simulink library "gm_ADC_Capture_4x4_IQ_DDR4_lib"  (R2019b)
settings: Solver=VariableStepAuto  StartTime=0.0  StopTime=10.0  RelTol=1e-3
undefined symbols (not defined in the file or in its folder): AXI4, Lite
libraries: axiinterfacelib x27
settings Model: Creator=larry  LastModifiedBy=larry

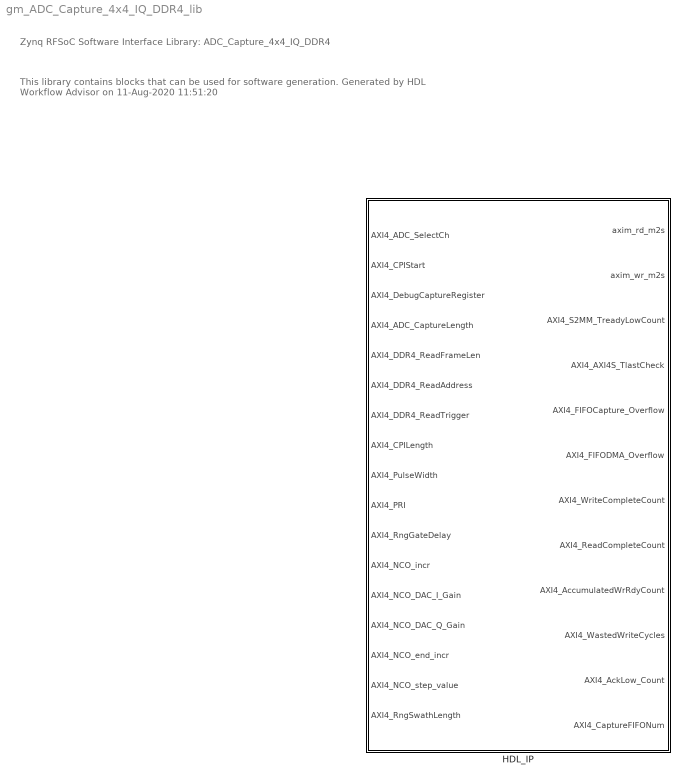
== system gm_ADC_Capture_4x4_IQ_DDR4_lib ==
  note: Zynq RFSoC Software Interface Library: ADC_Capture_4x4_IQ_DDR4
  note: This library contains blocks that can be used for software generation.
      |
      | Generated by HDL Workflow Advisor on 11-Aug-2020 11:51:20
  HDL_IP : Subsystem  TreatAsAtomicUnit=on  mask(AXI4-Lite/AXI4 Interface){}
      mask help:
      | This is an automatically generated subsystem block.
      | This contains the AXI interface blocks that communicate with the HDL_IP_ip IPCore generated from ADC_Capture_4x4_IQ_DDR4/HDL_IP subsystem.
      mask Display: disp(sprintf('Xilinx Zynq \nAXI Interface'));

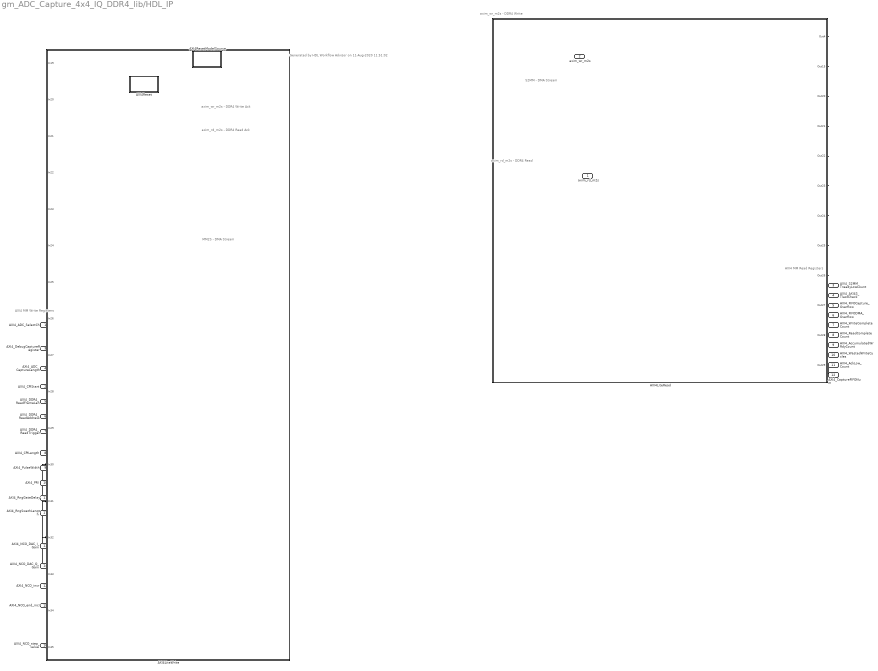
== system gm_ADC_Capture_4x4_IQ_DDR4_lib/HDL_IP ==
  note: Generated by HDL Workflow Advisor on 11-Aug-2020 11:51:02
  note: MM2S - DMA Stream
  note: axim_wr_m2s - DDR4 Write
  note: axim_rd_m2s - DDR4 Read Ack
  note: axim_rd_m2s - DDR4 Read
  note: axim_wr_m2s - DDR4 Write Ack
  note: S2MM - DMA Stream
  note: AXI4 MM Write Registers
  note: AXI4 MM Read Registers
  AXI4_ADC_SelectCh : Inport
  AXI4_CPIStart : Inport  Port=2
  AXI4_DebugCaptureRegister : Inport  Port=3
  AXI4_ADC_CaptureLength : Inport  Port=4
  AXI4_DDR4_ReadFrameLen : Inport  Port=5
  AXI4_DDR4_ReadAddress : Inport  Port=6
  AXI4_DDR4_ReadTrigger : Inport  Port=7
  AXI4_CPILength : Inport  Port=8
  AXI4_PulseWidth : Inport  Port=9
  AXI4_PRI : Inport  Port=10
  AXI4_RngGateDelay : Inport  Port=11
  AXI4_NCO_incr : Inport  Port=12
  AXI4_NCO_DAC_I_Gain : Inport  Port=13
  AXI4_NCO_DAC_Q_Gain : Inport  Port=14
  AXI4_NCO_end_incr : Inport  Port=15
  AXI4_NCO_step_value : Inport  Port=16
  AXI4_RngSwathLength : Inport  Port=17
  AXI4LiteRead : Subsystem  Priority=10
  AXI4LiteWrite : Subsystem  Priority=1
  AXI4Reset : Subsystem  mask(System Start){ShowInLibBrowser=0}
      mask prompts: ShowInLibBrowser "Simulink:masks:CustCodeMaskParam1_MP"
      settings: CopyFcn=cccopyfcn(gcb)  OpenFcn=ccopenfcn('System Start Function')
      mask Help: eval('feval(''rtwprivate'',''rtwhelpview'',''rtw_sys_start_block'')');
      mask Display: disp('System\nStart');
  AXI4ResetModelSource : Subsystem  mask(Model Source){ShowInLibBrowser=0}
      mask prompts: ShowInLibBrowser "Simulink:masks:CustCodeMaskParam1_MP"
      settings: CopyFcn=cccopyfcn(gcb)  OpenFcn=ccopenfcn('Model Source')
      mask Help: eval('feval(''rtwprivate'',''rtwhelpview'',''rtw_model_source_block'')');
      mask Display: disp('Model\nSource');
  axim_rd_m2s : Outport  VectorParamsAs1DForOutWhenUnconnected=off
  axim_wr_m2s : Outport  Port=2  VectorParamsAs1DForOutWhenUnconnected=off
  AXI4_S2MM_TreadyLowCount : Outport  Port=3  VectorParamsAs1DForOutWhenUnconnected=off
  AXI4_AXI4S_TlastCheck : Outport  Port=4  VectorParamsAs1DForOutWhenUnconnected=off
  AXI4_FIFOCapture_Overflow : Outport  Port=5  VectorParamsAs1DForOutWhenUnconnected=off
  AXI4_FIFODMA_Overflow : Outport  Port=6  VectorParamsAs1DForOutWhenUnconnected=off
  AXI4_WriteCompleteCount : Outport  Port=7  VectorParamsAs1DForOutWhenUnconnected=off
  AXI4_ReadCompleteCount : Outport  Port=8  VectorParamsAs1DForOutWhenUnconnected=off
  AXI4_AccumulatedWrRdyCount : Outport  Port=9  VectorParamsAs1DForOutWhenUnconnected=off
  AXI4_WastedWriteCycles : Outport  Port=10  VectorParamsAs1DForOutWhenUnconnected=off
  AXI4_AckLow_Count : Outport  Port=11  VectorParamsAs1DForOutWhenUnconnected=off
  AXI4_CaptureFIFONum : Outport  Port=12  VectorParamsAs1DForOutWhenUnconnected=off
  wires:
  AXI4LiteRead/12(Out29) -> AXI4_CaptureFIFONum/1
  AXI4LiteRead/11(Out28) -> AXI4_AckLow_Count/1
  AXI4LiteRead/10(Out27) -> AXI4_WastedWriteCycles/1
  AXI4LiteRead/9(Out26) -> AXI4_AccumulatedWrRdyCount/1
  AXI4LiteRead/8(Out25) -> AXI4_ReadCompleteCount/1
  AXI4LiteRead/7(Out24) -> AXI4_WriteCompleteCount/1
  AXI4LiteRead/6(Out23) -> AXI4_FIFODMA_Overflow/1
  AXI4LiteRead/5(Out22) -> AXI4_FIFOCapture_Overflow/1
  AXI4LiteRead/4(Out21) -> AXI4_AXI4S_TlastCheck/1
  AXI4LiteRead/3(Out20) -> AXI4_S2MM_TreadyLowCount/1
  AXI4LiteRead/2(Out15) -> axim_rd_m2s/1
  AXI4LiteRead/1(Out4) -> axim_wr_m2s/1
  AXI4_NCO_step_value/1 -> AXI4LiteWrite/17(In35)
  AXI4_NCO_end_incr/1 -> AXI4LiteWrite/16(In34)
  AXI4_NCO_incr/1 -> AXI4LiteWrite/15(In33)
  AXI4_NCO_DAC_Q_Gain/1 -> AXI4LiteWrite/14(In32)
  AXI4_NCO_DAC_I_Gain/1 -> AXI4LiteWrite/13(In31)
  AXI4_RngSwathLength/1 -> AXI4LiteWrite/12(In30)
  AXI4_RngGateDelay/1 -> AXI4LiteWrite/11(In29)
  AXI4_PRI/1 -> AXI4LiteWrite/10(In28)
  AXI4_PulseWidth/1 -> AXI4LiteWrite/9(In27)
  AXI4_CPILength/1 -> AXI4LiteWrite/8(In26)
  AXI4_DDR4_ReadTrigger/1 -> AXI4LiteWrite/7(In25)
  AXI4_DDR4_ReadAddress/1 -> AXI4LiteWrite/6(In24)
  AXI4_DDR4_ReadFrameLen/1 -> AXI4LiteWrite/5(In23)
  AXI4_CPIStart/1 -> AXI4LiteWrite/4(In22)
  AXI4_ADC_CaptureLength/1 -> AXI4LiteWrite/3(In21)
  AXI4_DebugCaptureRegister/1 -> AXI4LiteWrite/2(In20)
  AXI4_ADC_SelectCh/1 -> AXI4LiteWrite/1(In19)

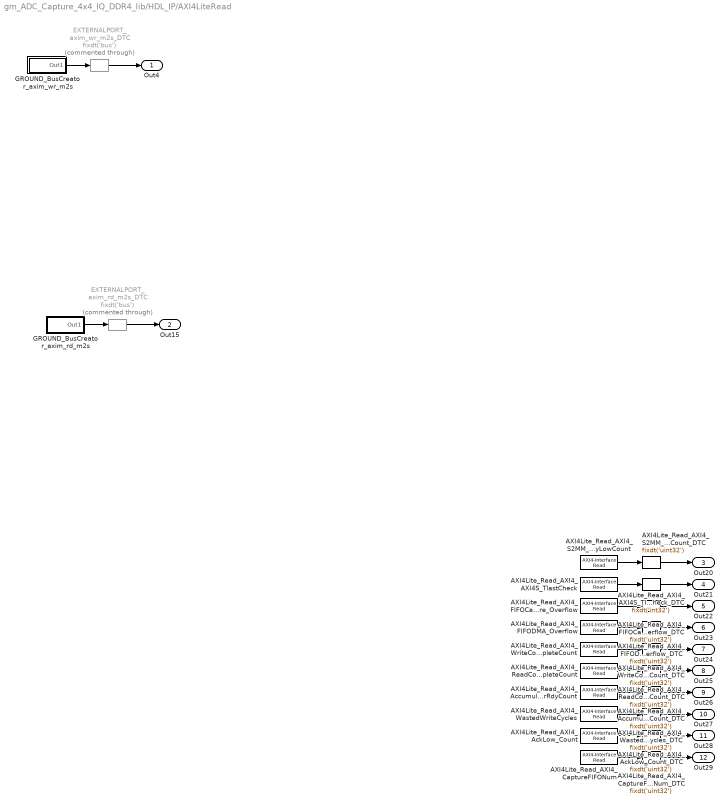
== system gm_ADC_Capture_4x4_IQ_DDR4_lib/HDL_IP/AXI4LiteRead ==
  AXI4Lite_Read_AXI4_AXI4S_TlastCheck : axiinterfacelib/AXI4-Interface Read  Priority=22  AXIInterfaceType=AXI4-Lite  DeviceName=/dev/mwipcore  RegisterOffset=hex2dec('148')  DataLength=1  DataType=uint32  SampleTime=-1  blockPlatform=ZYNQ  SimulateUsing=Interpreted Execution
      settings: SourceProductName=Embedded Coder Support Package for Xilinx Zynq Platform  SourceProductBaseCode=ECZYNQ7000
  AXI4Lite_Read_AXI4_AXI4S_TlastCheck_DTC : DataTypeConversion  OutDataTypeStr=fixdt('int32')  ConvertRealWorld=Stored Integer (SI)
  AXI4Lite_Read_AXI4_AccumulatedWrRdyCount : axiinterfacelib/AXI4-Interface Read  Priority=27  AXIInterfaceType=AXI4-Lite  DeviceName=/dev/mwipcore  RegisterOffset=hex2dec('15C')  DataLength=1  DataType=uint32  SampleTime=-1  blockPlatform=ZYNQ  SimulateUsing=Interpreted Execution
      settings: SourceProductName=Embedded Coder Support Package for Xilinx Zynq Platform  SourceProductBaseCode=ECZYNQ7000
  AXI4Lite_Read_AXI4_AccumulatedWrRdyCount_DTC : DataTypeConversion  OutDataTypeStr=fixdt('uint32')  ConvertRealWorld=Stored Integer (SI)
  AXI4Lite_Read_AXI4_AckLow_Count : axiinterfacelib/AXI4-Interface Read  Priority=29  AXIInterfaceType=AXI4-Lite  DeviceName=/dev/mwipcore  RegisterOffset=hex2dec('164')  DataLength=1  DataType=uint32  SampleTime=-1  blockPlatform=ZYNQ  SimulateUsing=Interpreted Execution
      settings: SourceProductName=Embedded Coder Support Package for Xilinx Zynq Platform  SourceProductBaseCode=ECZYNQ7000
  AXI4Lite_Read_AXI4_AckLow_Count_DTC : DataTypeConversion  OutDataTypeStr=fixdt('uint32')  ConvertRealWorld=Stored Integer (SI)
  AXI4Lite_Read_AXI4_CaptureFIFONum : axiinterfacelib/AXI4-Interface Read  Priority=30  AXIInterfaceType=AXI4-Lite  DeviceName=/dev/mwipcore  RegisterOffset=hex2dec('168')  DataLength=1  DataType=uint32  SampleTime=-1  blockPlatform=ZYNQ  SimulateUsing=Interpreted Execution
      settings: SourceProductName=Embedded Coder Support Package for Xilinx Zynq Platform  SourceProductBaseCode=ECZYNQ7000
  AXI4Lite_Read_AXI4_CaptureFIFONum_DTC : DataTypeConversion  OutDataTypeStr=fixdt('uint32')  ConvertRealWorld=Stored Integer (SI)
  AXI4Lite_Read_AXI4_FIFOCapture_Overflow : axiinterfacelib/AXI4-Interface Read  Priority=23  AXIInterfaceType=AXI4-Lite  DeviceName=/dev/mwipcore  RegisterOffset=hex2dec('14C')  DataLength=1  DataType=uint32  SampleTime=-1  blockPlatform=ZYNQ  SimulateUsing=Interpreted Execution
      settings: SourceProductName=Embedded Coder Support Package for Xilinx Zynq Platform  SourceProductBaseCode=ECZYNQ7000
  AXI4Lite_Read_AXI4_FIFOCapture_Overflow_DTC : DataTypeConversion  OutDataTypeStr=fixdt('uint32')  ConvertRealWorld=Stored Integer (SI)
  AXI4Lite_Read_AXI4_FIFODMA_Overflow : axiinterfacelib/AXI4-Interface Read  Priority=24  AXIInterfaceType=AXI4-Lite  DeviceName=/dev/mwipcore  RegisterOffset=hex2dec('150')  DataLength=1  DataType=uint32  SampleTime=-1  blockPlatform=ZYNQ  SimulateUsing=Interpreted Execution
      settings: SourceProductName=Embedded Coder Support Package for Xilinx Zynq Platform  SourceProductBaseCode=ECZYNQ7000
  AXI4Lite_Read_AXI4_FIFODMA_Overflow_DTC : DataTypeConversion  OutDataTypeStr=fixdt('uint32')  ConvertRealWorld=Stored Integer (SI)
  AXI4Lite_Read_AXI4_ReadCompleteCount : axiinterfacelib/AXI4-Interface Read  Priority=26  AXIInterfaceType=AXI4-Lite  DeviceName=/dev/mwipcore  RegisterOffset=hex2dec('158')  DataLength=1  DataType=uint32  SampleTime=-1  blockPlatform=ZYNQ  SimulateUsing=Interpreted Execution
      settings: SourceProductName=Embedded Coder Support Package for Xilinx Zynq Platform  SourceProductBaseCode=ECZYNQ7000
  AXI4Lite_Read_AXI4_ReadCompleteCount_DTC : DataTypeConversion  OutDataTypeStr=fixdt('uint32')  ConvertRealWorld=Stored Integer (SI)
  AXI4Lite_Read_AXI4_S2MM_TreadyLowCount : axiinterfacelib/AXI4-Interface Read  Priority=21  AXIInterfaceType=AXI4-Lite  DeviceName=/dev/mwipcore  RegisterOffset=hex2dec('144')  DataLength=1  DataType=uint32  SampleTime=-1  blockPlatform=ZYNQ  SimulateUsing=Interpreted Execution
      settings: SourceProductName=Embedded Coder Support Package for Xilinx Zynq Platform  SourceProductBaseCode=ECZYNQ7000
  AXI4Lite_Read_AXI4_S2MM_TreadyLowCount_DTC : DataTypeConversion  OutDataTypeStr=fixdt('uint32')  ConvertRealWorld=Stored Integer (SI)
  AXI4Lite_Read_AXI4_WastedWriteCycles : axiinterfacelib/AXI4-Interface Read  Priority=28  AXIInterfaceType=AXI4-Lite  DeviceName=/dev/mwipcore  RegisterOffset=hex2dec('160')  DataLength=1  DataType=uint32  SampleTime=-1  blockPlatform=ZYNQ  SimulateUsing=Interpreted Execution
      settings: SourceProductName=Embedded Coder Support Package for Xilinx Zynq Platform  SourceProductBaseCode=ECZYNQ7000
  AXI4Lite_Read_AXI4_WastedWriteCycles_DTC : DataTypeConversion  OutDataTypeStr=fixdt('uint32')  ConvertRealWorld=Stored Integer (SI)
  AXI4Lite_Read_AXI4_WriteCompleteCount : axiinterfacelib/AXI4-Interface Read  Priority=25  AXIInterfaceType=AXI4-Lite  DeviceName=/dev/mwipcore  RegisterOffset=hex2dec('154')  DataLength=1  DataType=uint32  SampleTime=-1  blockPlatform=ZYNQ  SimulateUsing=Interpreted Execution
      settings: SourceProductName=Embedded Coder Support Package for Xilinx Zynq Platform  SourceProductBaseCode=ECZYNQ7000
  AXI4Lite_Read_AXI4_WriteCompleteCount_DTC : DataTypeConversion  OutDataTypeStr=fixdt('uint32')  ConvertRealWorld=Stored Integer (SI)
  EXTERNALPORT_axim_rd_m2s_DTC : DataTypeConversion  Commented=through  OutDataTypeStr=fixdt('bus')
  EXTERNALPORT_axim_wr_m2s_DTC : DataTypeConversion  Commented=through  OutDataTypeStr=fixdt('bus')
  GROUND_BusCreator_axim_rd_m2s : Subsystem
  GROUND_BusCreator_axim_wr_m2s : Subsystem
  Out4 : Outport
  Out15 : Outport  Port=2
  Out20 : Outport  Port=3
  Out21 : Outport  Port=4
  Out22 : Outport  Port=5
  Out23 : Outport  Port=6
  Out24 : Outport  Port=7
  Out25 : Outport  Port=8
  Out26 : Outport  Port=9
  Out27 : Outport  Port=10
  Out28 : Outport  Port=11
  Out29 : Outport  Port=12
  wires:
  AXI4Lite_Read_AXI4_AckLow_Count_DTC/1 -> Out28/1
  EXTERNALPORT_axim_wr_m2s_DTC/1 -> Out4/1
  AXI4Lite_Read_AXI4_ReadCompleteCount_DTC/1 -> Out25/1
  AXI4Lite_Read_AXI4_WastedWriteCycles_DTC/1 -> Out27/1
  AXI4Lite_Read_AXI4_CaptureFIFONum_DTC/1 -> Out29/1
  AXI4Lite_Read_AXI4_AccumulatedWrRdyCount/1 -> AXI4Lite_Read_AXI4_AccumulatedWrRdyCount_DTC/1
  AXI4Lite_Read_AXI4_AckLow_Count/1 -> AXI4Lite_Read_AXI4_AckLow_Count_DTC/1
  AXI4Lite_Read_AXI4_AXI4S_TlastCheck/1 -> AXI4Lite_Read_AXI4_AXI4S_TlastCheck_DTC/1
  AXI4Lite_Read_AXI4_WriteCompleteCount/1 -> AXI4Lite_Read_AXI4_WriteCompleteCount_DTC/1
  AXI4Lite_Read_AXI4_S2MM_TreadyLowCount_DTC/1 -> Out20/1
  GROUND_BusCreator_axim_wr_m2s/1(Out1) -> EXTERNALPORT_axim_wr_m2s_DTC/1
  EXTERNALPORT_axim_rd_m2s_DTC/1 -> Out15/1
  AXI4Lite_Read_AXI4_WastedWriteCycles/1 -> AXI4Lite_Read_AXI4_WastedWriteCycles_DTC/1
  AXI4Lite_Read_AXI4_CaptureFIFONum/1 -> AXI4Lite_Read_AXI4_CaptureFIFONum_DTC/1
  AXI4Lite_Read_AXI4_FIFODMA_Overflow_DTC/1 -> Out23/1
  AXI4Lite_Read_AXI4_AXI4S_TlastCheck_DTC/1 -> Out21/1
  AXI4Lite_Read_AXI4_S2MM_TreadyLowCount/1 -> AXI4Lite_Read_AXI4_S2MM_TreadyLowCount_DTC/1
  AXI4Lite_Read_AXI4_AccumulatedWrRdyCount_DTC/1 -> Out26/1
  AXI4Lite_Read_AXI4_FIFOCapture_Overflow/1 -> AXI4Lite_Read_AXI4_FIFOCapture_Overflow_DTC/1
  AXI4Lite_Read_AXI4_ReadCompleteCount/1 -> AXI4Lite_Read_AXI4_ReadCompleteCount_DTC/1
  AXI4Lite_Read_AXI4_FIFOCapture_Overflow_DTC/1 -> Out22/1
  AXI4Lite_Read_AXI4_FIFODMA_Overflow/1 -> AXI4Lite_Read_AXI4_FIFODMA_Overflow_DTC/1
  AXI4Lite_Read_AXI4_WriteCompleteCount_DTC/1 -> Out24/1
  GROUND_BusCreator_axim_rd_m2s/1(Out1) -> EXTERNALPORT_axim_rd_m2s_DTC/1

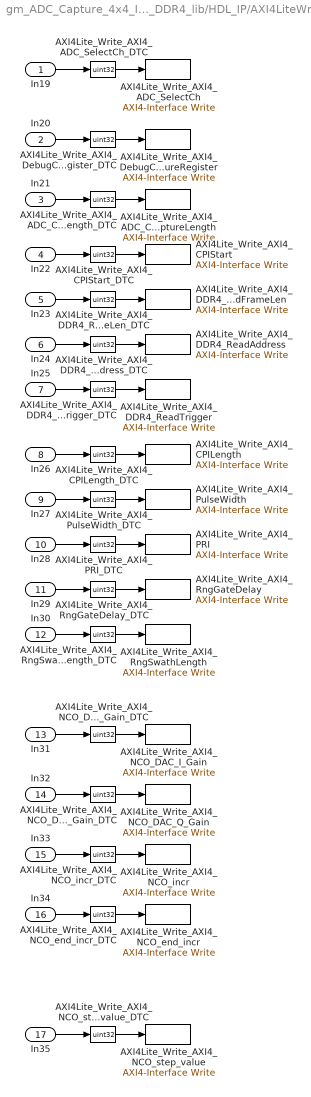
== system gm_ADC_Capture_4x4_IQ_DDR4_lib/HDL_IP/AXI4LiteWrite ==
  In19 : Inport
  In20 : Inport  Port=2
  In21 : Inport  Port=3
  In22 : Inport  Port=4
  In23 : Inport  Port=5
  In24 : Inport  Port=6
  In25 : Inport  Port=7
  In26 : Inport  Port=8
  In27 : Inport  Port=9
  In28 : Inport  Port=10
  In29 : Inport  Port=11
  In30 : Inport  Port=12
  In31 : Inport  Port=13
  In32 : Inport  Port=14
  In33 : Inport  Port=15
  In34 : Inport  Port=16
  In35 : Inport  Port=17
  AXI4Lite_Write_AXI4_ADC_CaptureLength : axiinterfacelib/AXI4-Interface Write  Priority=22  AXIInterfaceType=AXI4-Lite  DeviceName=/dev/mwipcore  RegisterOffset=hex2dec('104')  blockPlatform=ZYNQ  SimulateUsing=Interpreted execution
      settings: SourceProductName=Embedded Coder Support Package for Xilinx Zynq Platform  SourceProductBaseCode=ECZYNQ7000
  AXI4Lite_Write_AXI4_ADC_CaptureLength_DTC : DataTypeConversion  OutDataTypeStr=uint32  ConvertRealWorld=Stored Integer (SI)
  AXI4Lite_Write_AXI4_ADC_SelectCh : axiinterfacelib/AXI4-Interface Write  Priority=19  AXIInterfaceType=AXI4-Lite  DeviceName=/dev/mwipcore  RegisterOffset=hex2dec('11C')  blockPlatform=ZYNQ  SimulateUsing=Interpreted execution
      settings: SourceProductName=Embedded Coder Support Package for Xilinx Zynq Platform  SourceProductBaseCode=ECZYNQ7000
  AXI4Lite_Write_AXI4_ADC_SelectCh_DTC : DataTypeConversion  OutDataTypeStr=uint32  ConvertRealWorld=Stored Integer (SI)
  AXI4Lite_Write_AXI4_CPILength : axiinterfacelib/AXI4-Interface Write  Priority=26  AXIInterfaceType=AXI4-Lite  DeviceName=/dev/mwipcore  RegisterOffset=hex2dec('120')  blockPlatform=ZYNQ  SimulateUsing=Interpreted execution
      settings: SourceProductName=Embedded Coder Support Package for Xilinx Zynq Platform  SourceProductBaseCode=ECZYNQ7000
  AXI4Lite_Write_AXI4_CPILength_DTC : DataTypeConversion  OutDataTypeStr=uint32  ConvertRealWorld=Stored Integer (SI)
  AXI4Lite_Write_AXI4_CPIStart : axiinterfacelib/AXI4-Interface Write  Priority=20  AXIInterfaceType=AXI4-Lite  DeviceName=/dev/mwipcore  RegisterOffset=hex2dec('100')  blockPlatform=ZYNQ  SimulateUsing=Interpreted execution
      settings: SourceProductName=Embedded Coder Support Package for Xilinx Zynq Platform  SourceProductBaseCode=ECZYNQ7000
  AXI4Lite_Write_AXI4_CPIStart_DTC : DataTypeConversion  OutDataTypeStr=uint32  ConvertRealWorld=Stored Integer (SI)
  AXI4Lite_Write_AXI4_DDR4_ReadAddress : axiinterfacelib/AXI4-Interface Write  Priority=24  AXIInterfaceType=AXI4-Lite  DeviceName=/dev/mwipcore  RegisterOffset=hex2dec('110')  blockPlatform=ZYNQ  SimulateUsing=Interpreted execution
      settings: SourceProductName=Embedded Coder Support Package for Xilinx Zynq Platform  SourceProductBaseCode=ECZYNQ7000
  AXI4Lite_Write_AXI4_DDR4_ReadAddress_DTC : DataTypeConversion  OutDataTypeStr=uint32  ConvertRealWorld=Stored Integer (SI)
  AXI4Lite_Write_AXI4_DDR4_ReadFrameLen : axiinterfacelib/AXI4-Interface Write  Priority=23  AXIInterfaceType=AXI4-Lite  DeviceName=/dev/mwipcore  RegisterOffset=hex2dec('10C')  blockPlatform=ZYNQ  SimulateUsing=Interpreted execution
      settings: SourceProductName=Embedded Coder Support Package for Xilinx Zynq Platform  SourceProductBaseCode=ECZYNQ7000
  AXI4Lite_Write_AXI4_DDR4_ReadFrameLen_DTC : DataTypeConversion  OutDataTypeStr=uint32  ConvertRealWorld=Stored Integer (SI)
  AXI4Lite_Write_AXI4_DDR4_ReadTrigger : axiinterfacelib/AXI4-Interface Write  Priority=25  AXIInterfaceType=AXI4-Lite  DeviceName=/dev/mwipcore  RegisterOffset=hex2dec('114')  blockPlatform=ZYNQ  SimulateUsing=Interpreted execution
      settings: SourceProductName=Embedded Coder Support Package for Xilinx Zynq Platform  SourceProductBaseCode=ECZYNQ7000
  AXI4Lite_Write_AXI4_DDR4_ReadTrigger_DTC : DataTypeConversion  OutDataTypeStr=uint32  ConvertRealWorld=Stored Integer (SI)
  AXI4Lite_Write_AXI4_DebugCaptureRegister : axiinterfacelib/AXI4-Interface Write  Priority=21  AXIInterfaceType=AXI4-Lite  DeviceName=/dev/mwipcore  RegisterOffset=hex2dec('108')  blockPlatform=ZYNQ  SimulateUsing=Interpreted execution
      settings: SourceProductName=Embedded Coder Support Package for Xilinx Zynq Platform  SourceProductBaseCode=ECZYNQ7000
  AXI4Lite_Write_AXI4_DebugCaptureRegister_DTC : DataTypeConversion  OutDataTypeStr=uint32  ConvertRealWorld=Stored Integer (SI)
  AXI4Lite_Write_AXI4_NCO_DAC_I_Gain : axiinterfacelib/AXI4-Interface Write  Priority=31  AXIInterfaceType=AXI4-Lite  DeviceName=/dev/mwipcore  RegisterOffset=hex2dec('130')  blockPlatform=ZYNQ  SimulateUsing=Interpreted execution
      settings: SourceProductName=Embedded Coder Support Package for Xilinx Zynq Platform  SourceProductBaseCode=ECZYNQ7000
  AXI4Lite_Write_AXI4_NCO_DAC_I_Gain_DTC : DataTypeConversion  OutDataTypeStr=uint32  ConvertRealWorld=Stored Integer (SI)
  AXI4Lite_Write_AXI4_NCO_DAC_Q_Gain : axiinterfacelib/AXI4-Interface Write  Priority=32  AXIInterfaceType=AXI4-Lite  DeviceName=/dev/mwipcore  RegisterOffset=hex2dec('134')  blockPlatform=ZYNQ  SimulateUsing=Interpreted execution
      settings: SourceProductName=Embedded Coder Support Package for Xilinx Zynq Platform  SourceProductBaseCode=ECZYNQ7000
  AXI4Lite_Write_AXI4_NCO_DAC_Q_Gain_DTC : DataTypeConversion  OutDataTypeStr=uint32  ConvertRealWorld=Stored Integer (SI)
  AXI4Lite_Write_AXI4_NCO_end_incr : axiinterfacelib/AXI4-Interface Write  Priority=33  AXIInterfaceType=AXI4-Lite  DeviceName=/dev/mwipcore  RegisterOffset=hex2dec('138')  blockPlatform=ZYNQ  SimulateUsing=Interpreted execution
      settings: SourceProductName=Embedded Coder Support Package for Xilinx Zynq Platform  SourceProductBaseCode=ECZYNQ7000
  AXI4Lite_Write_AXI4_NCO_end_incr_DTC : DataTypeConversion  OutDataTypeStr=uint32  ConvertRealWorld=Stored Integer (SI)
  AXI4Lite_Write_AXI4_NCO_incr : axiinterfacelib/AXI4-Interface Write  Priority=30  AXIInterfaceType=AXI4-Lite  DeviceName=/dev/mwipcore  RegisterOffset=hex2dec('118')  blockPlatform=ZYNQ  SimulateUsing=Interpreted execution
      settings: SourceProductName=Embedded Coder Support Package for Xilinx Zynq Platform  SourceProductBaseCode=ECZYNQ7000
  AXI4Lite_Write_AXI4_NCO_incr_DTC : DataTypeConversion  OutDataTypeStr=uint32  ConvertRealWorld=Stored Integer (SI)
  AXI4Lite_Write_AXI4_NCO_step_value : axiinterfacelib/AXI4-Interface Write  Priority=34  AXIInterfaceType=AXI4-Lite  DeviceName=/dev/mwipcore  RegisterOffset=hex2dec('140')  blockPlatform=ZYNQ  SimulateUsing=Interpreted execution
      settings: SourceProductName=Embedded Coder Support Package for Xilinx Zynq Platform  SourceProductBaseCode=ECZYNQ7000
  AXI4Lite_Write_AXI4_NCO_step_value_DTC : DataTypeConversion  OutDataTypeStr=uint32  ConvertRealWorld=Stored Integer (SI)
  AXI4Lite_Write_AXI4_PRI : axiinterfacelib/AXI4-Interface Write  Priority=28  AXIInterfaceType=AXI4-Lite  DeviceName=/dev/mwipcore  RegisterOffset=hex2dec('128')  blockPlatform=ZYNQ  SimulateUsing=Interpreted execution
      settings: SourceProductName=Embedded Coder Support Package for Xilinx Zynq Platform  SourceProductBaseCode=ECZYNQ7000
  AXI4Lite_Write_AXI4_PRI_DTC : DataTypeConversion  OutDataTypeStr=uint32  ConvertRealWorld=Stored Integer (SI)
  AXI4Lite_Write_AXI4_PulseWidth : axiinterfacelib/AXI4-Interface Write  Priority=27  AXIInterfaceType=AXI4-Lite  DeviceName=/dev/mwipcore  RegisterOffset=hex2dec('124')  blockPlatform=ZYNQ  SimulateUsing=Interpreted execution
      settings: SourceProductName=Embedded Coder Support Package for Xilinx Zynq Platform  SourceProductBaseCode=ECZYNQ7000
  AXI4Lite_Write_AXI4_PulseWidth_DTC : DataTypeConversion  OutDataTypeStr=uint32  ConvertRealWorld=Stored Integer (SI)
  AXI4Lite_Write_AXI4_RngGateDelay : axiinterfacelib/AXI4-Interface Write  Priority=29  AXIInterfaceType=AXI4-Lite  DeviceName=/dev/mwipcore  RegisterOffset=hex2dec('12C')  blockPlatform=ZYNQ  SimulateUsing=Interpreted execution
      settings: SourceProductName=Embedded Coder Support Package for Xilinx Zynq Platform  SourceProductBaseCode=ECZYNQ7000
  AXI4Lite_Write_AXI4_RngGateDelay_DTC : DataTypeConversion  OutDataTypeStr=uint32  ConvertRealWorld=Stored Integer (SI)
  AXI4Lite_Write_AXI4_RngSwathLength : axiinterfacelib/AXI4-Interface Write  Priority=35  AXIInterfaceType=AXI4-Lite  DeviceName=/dev/mwipcore  RegisterOffset=hex2dec('13C')  blockPlatform=ZYNQ  SimulateUsing=Interpreted execution
      settings: SourceProductName=Embedded Coder Support Package for Xilinx Zynq Platform  SourceProductBaseCode=ECZYNQ7000
  AXI4Lite_Write_AXI4_RngSwathLength_DTC : DataTypeConversion  OutDataTypeStr=uint32  ConvertRealWorld=Stored Integer (SI)
  wires:
  In29/1 -> AXI4Lite_Write_AXI4_RngGateDelay_DTC/1
  In32/1 -> AXI4Lite_Write_AXI4_NCO_DAC_Q_Gain_DTC/1
  In19/1 -> AXI4Lite_Write_AXI4_ADC_SelectCh_DTC/1
  In34/1 -> AXI4Lite_Write_AXI4_NCO_end_incr_DTC/1
  In35/1 -> AXI4Lite_Write_AXI4_NCO_step_value_DTC/1
  In21/1 -> AXI4Lite_Write_AXI4_ADC_CaptureLength_DTC/1
  In28/1 -> AXI4Lite_Write_AXI4_PRI_DTC/1
  In31/1 -> AXI4Lite_Write_AXI4_NCO_DAC_I_Gain_DTC/1
  AXI4Lite_Write_AXI4_DDR4_ReadTrigger_DTC/1 -> AXI4Lite_Write_AXI4_DDR4_ReadTrigger/1
  In25/1 -> AXI4Lite_Write_AXI4_DDR4_ReadTrigger_DTC/1
  AXI4Lite_Write_AXI4_PulseWidth_DTC/1 -> AXI4Lite_Write_AXI4_PulseWidth/1
  AXI4Lite_Write_AXI4_RngGateDelay_DTC/1 -> AXI4Lite_Write_AXI4_RngGateDelay/1
  In24/1 -> AXI4Lite_Write_AXI4_DDR4_ReadAddress_DTC/1
  In33/1 -> AXI4Lite_Write_AXI4_NCO_incr_DTC/1
  AXI4Lite_Write_AXI4_ADC_SelectCh_DTC/1 -> AXI4Lite_Write_AXI4_ADC_SelectCh/1
  In20/1 -> AXI4Lite_Write_AXI4_DebugCaptureRegister_DTC/1
  In23/1 -> AXI4Lite_Write_AXI4_DDR4_ReadFrameLen_DTC/1
  In27/1 -> AXI4Lite_Write_AXI4_PulseWidth_DTC/1
  AXI4Lite_Write_AXI4_NCO_DAC_Q_Gain_DTC/1 -> AXI4Lite_Write_AXI4_NCO_DAC_Q_Gain/1
  AXI4Lite_Write_AXI4_RngSwathLength_DTC/1 -> AXI4Lite_Write_AXI4_RngSwathLength/1
  AXI4Lite_Write_AXI4_DebugCaptureRegister_DTC/1 -> AXI4Lite_Write_AXI4_DebugCaptureRegister/1
  AXI4Lite_Write_AXI4_NCO_step_value_DTC/1 -> AXI4Lite_Write_AXI4_NCO_step_value/1
  AXI4Lite_Write_AXI4_NCO_end_incr_DTC/1 -> AXI4Lite_Write_AXI4_NCO_end_incr/1
  In22/1 -> AXI4Lite_Write_AXI4_CPIStart_DTC/1
  AXI4Lite_Write_AXI4_NCO_incr_DTC/1 -> AXI4Lite_Write_AXI4_NCO_incr/1
  AXI4Lite_Write_AXI4_ADC_CaptureLength_DTC/1 -> AXI4Lite_Write_AXI4_ADC_CaptureLength/1
  AXI4Lite_Write_AXI4_DDR4_ReadAddress_DTC/1 -> AXI4Lite_Write_AXI4_DDR4_ReadAddress/1
  AXI4Lite_Write_AXI4_DDR4_ReadFrameLen_DTC/1 -> AXI4Lite_Write_AXI4_DDR4_ReadFrameLen/1
  AXI4Lite_Write_AXI4_PRI_DTC/1 -> AXI4Lite_Write_AXI4_PRI/1
  In30/1 -> AXI4Lite_Write_AXI4_RngSwathLength_DTC/1
  AXI4Lite_Write_AXI4_CPILength_DTC/1 -> AXI4Lite_Write_AXI4_CPILength/1
  AXI4Lite_Write_AXI4_CPIStart_DTC/1 -> AXI4Lite_Write_AXI4_CPIStart/1
  In26/1 -> AXI4Lite_Write_AXI4_CPILength_DTC/1
  AXI4Lite_Write_AXI4_NCO_DAC_I_Gain_DTC/1 -> AXI4Lite_Write_AXI4_NCO_DAC_I_Gain/1

== system gm_ADC_Capture_4x4_IQ_DDR4_lib/HDL_IP/AXI4Reset ==

== system gm_ADC_Capture_4x4_IQ_DDR4_lib/HDL_IP/AXI4ResetModelSource ==

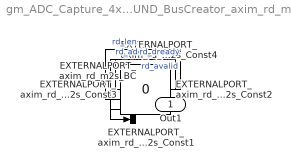
== system gm_ADC_Capture_4x4_IQ_DDR4_lib/HDL_IP/AXI4LiteRead/GROUND_BusCreator_axim_rd_m2s ==
  EXTERNALPORT_axim_rd_m2s_BC : BusCreator  Inputs=4
  EXTERNALPORT_axim_rd_m2s_Const1 : Constant  Value=0  OutDataTypeStr=fixdt(0,32,0)  SampleTime=-1
  EXTERNALPORT_axim_rd_m2s_Const2 : Constant  Value=0  OutDataTypeStr=fixdt(0,32,0)  SampleTime=-1
  EXTERNALPORT_axim_rd_m2s_Const3 : Constant  Value=0  OutDataTypeStr=fixdt('boolean')  SampleTime=-1
  EXTERNALPORT_axim_rd_m2s_Const4 : Constant  Value=0  OutDataTypeStr=fixdt('boolean')  SampleTime=-1
  Out1 : Outport
  wires:
  EXTERNALPORT_axim_rd_m2s_Const3/1 -> EXTERNALPORT_axim_rd_m2s_BC/3  "rd_avalid"
  EXTERNALPORT_axim_rd_m2s_Const1/1 -> EXTERNALPORT_axim_rd_m2s_BC/1  "rd_addr"
  EXTERNALPORT_axim_rd_m2s_Const2/1 -> EXTERNALPORT_axim_rd_m2s_BC/2  "rd_len"
  EXTERNALPORT_axim_rd_m2s_BC/1 -> Out1/1
  EXTERNALPORT_axim_rd_m2s_Const4/1 -> EXTERNALPORT_axim_rd_m2s_BC/4  "rd_dready"

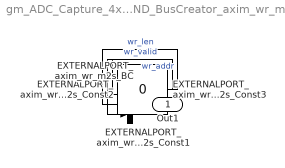
== system gm_ADC_Capture_4x4_IQ_DDR4_lib/HDL_IP/AXI4LiteRead/GROUND_BusCreator_axim_wr_m2s ==
  EXTERNALPORT_axim_wr_m2s_BC : BusCreator  Inputs=3
  EXTERNALPORT_axim_wr_m2s_Const1 : Constant  Value=0  OutDataTypeStr=fixdt(0,32,0)  SampleTime=-1
  EXTERNALPORT_axim_wr_m2s_Const2 : Constant  Value=0  OutDataTypeStr=fixdt(0,32,0)  SampleTime=-1
  EXTERNALPORT_axim_wr_m2s_Const3 : Constant  Value=0  OutDataTypeStr=fixdt('boolean')  SampleTime=-1
  Out1 : Outport
  wires:
  EXTERNALPORT_axim_wr_m2s_BC/1 -> Out1/1
  EXTERNALPORT_axim_wr_m2s_Const2/1 -> EXTERNALPORT_axim_wr_m2s_BC/2  "wr_len"
  EXTERNALPORT_axim_wr_m2s_Const3/1 -> EXTERNALPORT_axim_wr_m2s_BC/3  "wr_valid"
  EXTERNALPORT_axim_wr_m2s_Const1/1 -> EXTERNALPORT_axim_wr_m2s_BC/1  "wr_addr"
